simulink model "ekviv_prenos_nelin_1"  (R2018a)
settings: Solver=VariableStepAuto  StartTime=0.0  StopTime=10.0  RelTol=1e-3
undefined symbols (not defined in the file or in its folder): toff, ton
settings Model: Creator=vejvarm  LastModifiedBy=vejvarm

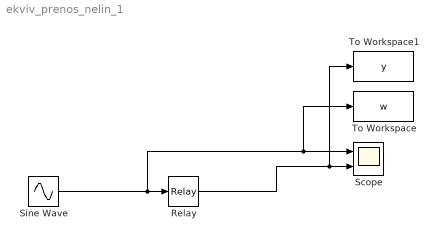
== system ekviv_prenos_nelin_1 ==
  Relay : Relay  OnSwitchValue=ton  OffSwitchValue=toff  OnOutputValue=Mon  OffOutputValue=Moff
  Scope : Scope  NumInputPorts=2
  Sine Wave : Sin  Amplitude=2  Frequency=2  SampleTime=0
  To Workspace : ToWorkspace  VariableName=w  SaveFormat=Timeseries  SampleTime=-1
  To Workspace1 : ToWorkspace  VariableName=y  SaveFormat=Timeseries  SampleTime=-1
  wires:
  Relay/1 -> To Workspace1/1, Scope/2
  Sine Wave/1 -> Relay/1, To Workspace/1, Scope/1
